simulink model "pen_sim"  (R2017a)
settings: Solver=VariableStepAuto  StartTime=0.0  StopTime=10.0  RelTol=1e-3  EnableMultiTasking=on
values from neighbouring files (symbols this model uses):
  c = P(2)*m*g*l    [Lab2_2.m]
  g = 9.8    [Lab2_2.m]
  l = P(1)*g    [Lab2_2.m]
  m = 0.2    [Lab2_2.m]
settings Model: Creator=c3204612  LastModifiedBy=Administrator
settings DataIOCC: InitialState=[1.1, 0]  LimitDataPoints=on  LoadInitialState=on
settings OptimizationCC: LifeSpan=inf
settings DebuggingCC: AllowSymbolicDim=off  SFUnexpectedBacktrackingDiag=warning  SFNoUnconditionalDefaultTransitionDiag=warning  SFExecutionAtInitializationDiag=none
settings ModelReferenceCC: PropagateSignalLabelsOutOfModel=off
settings GRTTargetCC: TargetLangStandard=C89/C90 (ANSI)
settings ConfigComp: CovMetricSettings=dw  CovHtmlReporting=on  CovSaveCumulativeToWorkspaceVar=on  CovSaveSingleToWorkspaceVar=on  CovExternalEMLEnable=off

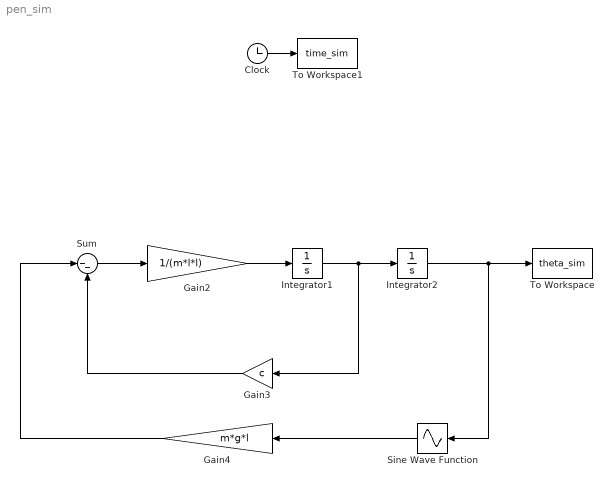
== system pen_sim ==
  Clock : Clock
  Gain2 : Gain  Gain=1/(m*l*l)
  Gain3 : Gain  Gain=c
  Gain4 : Gain  Gain=m*g*l
  Integrator1 : Integrator
  Integrator2 : Integrator
  Sine Wave Function : Sin  TimeSource=Use external signal  SampleTime=0
  Sum : Sum  Inputs=|--
  To Workspace : ToWorkspace  VariableName=theta_sim  SampleTime=-1
  To Workspace1 : ToWorkspace  VariableName=time_sim  SampleTime=-1
  wires:
  Gain2/1 -> Integrator1/1
  Sine Wave Function/1 -> Gain4/1
  Gain3/1 -> Sum/2
  Integrator1/1 -> Gain3/1, Integrator2/1
  Integrator2/1 -> To Workspace/1, Sine Wave Function/1
  Clock/1 -> To Workspace1/1
  Gain4/1 -> Sum/1
  Sum/1 -> Gain2/1
